simulink model "sf_fixpt"  (Simulink 7.6)
settings: Solver=ode45  StartTime=0.0  StopTime=1  RelTol=1e-3
settings Model: Creator=The MathWorks Inc.  CovMetricSettings=dcmtr  ExtModeAutoUpdateStatusClock=off
settings DataIOCC: SignalLoggingName=sigsOut
settings OptimizationCC: InlineInvariantSignals=on  InitFltsAndDblsToZero=on  EfficientMapNaN2IntZero=off
settings DebuggingCC: SaveWithParameterizedLinksMsg=none  SignalResolutionControl=TryResolveAllWithWarning  SolverPrmCheckMsg=none  MultiTaskDSMMsg=warning  MultiTaskCondExecSysMsg=none  StrictBusMsg=None
settings HardwareCC: TargetUnknown=on
settings SFSimCC: SimParseCustomCode=off
settings RTWCC: IncludeERTFirstTime=on
settings GRTTargetCC: TargetFcnLib=ansi_tfl_tmw.mat

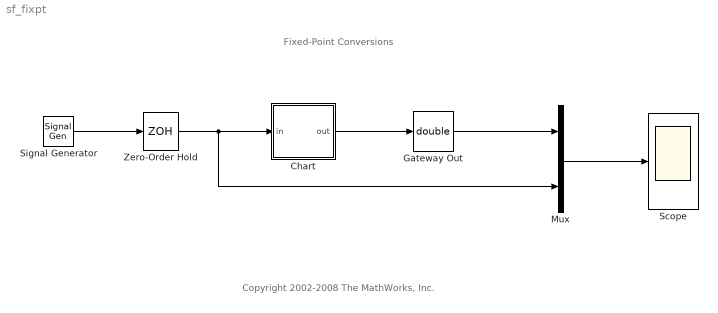
== system sf_fixpt ==
  note: Fixed-Point Conversions
  note: Copyright 2002-2008 The MathWorks, Inc.
  Chart : Stateflow chart  TreatAsAtomicUnit=on
  Gateway Out : DataTypeConversion  OutDataTypeStr=double
  Mux : Mux  Inputs=2
  Scope : Scope
      settings: TimeRange=1  YMin=-10  YMax=10
  Signal Generator : SignalGenerator  WaveForm=sawtooth  Amplitude=10
  Zero-Order Hold : ZeroOrderHold  SampleTime=.001
  wires:
  Chart/1(out) -> Gateway Out/1
  Signal Generator/1 -> Zero-Order Hold/1
  Zero-Order Hold/1 -> Chart/1(in), Mux/2
  Gateway Out/1 -> Mux/1
  Mux/1 -> Scope/1

== stateflow chart Chart ==
  note: Note: Converting a double to a fixpt type
      | contains an inherent overflow and this
      | is detected by the Stateflow Debugger.
      | For illustrative purposes, this data-range
      | check is turned off in the Stateflow Debugger.
  (default) -> (junction 4) : {out=in;}
  data: in input double; out output fixdt(1,8,5)
